simulink model "power_wind_dfig"  (R2016a)
settings: Solver=ode23tb  StartTime=0.0  StopTime=100  FixedStep=1/60  MaxStep=1/60  RelTol=1e-4  AbsTol=1e-3
InitFcn:
  | xInitial = init_power_wind_dfig;
undefined symbols (not defined in the file): b0, D1, D11, Delta, F, find_system, Fnom, gcbh, H, ILd_init, ILq_init, Imax_grid_conv, Init, j, Kd, Ki_dc_reg, Ki_grid_side_cur_reg, Ki_power_reg, Ki_Q, Ki_rotor_side_cur_reg, Ki_volt_reg, Kp, Kp_dc_reg, Kp_grid_side_cur_reg, Kp_power_reg, Kp_Q, Kp_rotor_side_cur_reg, Kp_volt_reg, L_RL, Llr, Lls, p, Pnom, power_A, power_B, power_D, R_RL, Rr, Rs, speed_A, speed_B, speed_C, speed_D, sps_rtmsupport, Vcontrol, Vnom, Wind_On, wo
libraries: powerlib_meascontrol x29, powerlib x27, simulink_extras x5, re_lib x2
(part 1 of 5)
Description:
  | Copyright 2008-2016 The MathWorks, Inc.
settings Model: ExtModeAutoUpdateStatusClock=off  Creator=MathWorks  LastModifiedBy=farhan an
settings DataIOCC: LimitDataPoints=on  LoadInitialState=on  SaveFormat=StructureWithTime  SignalLoggingSaveFormat=ModelDataLogs  SaveOutput=off  InspectSignalLogs=on  SaveTime=off  SignalLoggingName=sigsOut
settings OptimizationCC: ExpressionDepthLimit=2147483647  InitFltsAndDblsToZero=on  EfficientMapNaN2IntZero=off
settings DebuggingCC: UnderspecifiedInitializationDetection=Classic  MergeDetectMultiDrivingBlocksExec=none  CheckExecutionContextPreStartOutputMsg=on  CheckExecutionContextRuntimeOutputMsg=on  SignalResolutionControl=TryResolveAllWithWarning  MultiTaskDSMMsg=warning  MultiTaskCondExecSysMsg=none  FcnCallInpInsideContextMsg=UseLocalSettings  UnconnectedLineMsg=none  StateNameClashWarn=warning  InitInArrayFormatMsg=none
settings HardwareCC: ProdBitPerPointer=32  ProdLargestAtomicFloat=None  ProdIntDivRoundTo=Undefined  ProdEndianess=Unspecified  ProdWordSize=32  ProdHWDeviceType=32-bit Generic  TargetUnknown=on
settings ModelReferenceCC: PropagateSignalLabelsOutOfModel=off
settings GRTTargetCC: CombineOutputUpdateFcns=off  GRTInterface=on
settings ConfigComp: CovModelRefEnable=Off  CovSFcnEnable=off

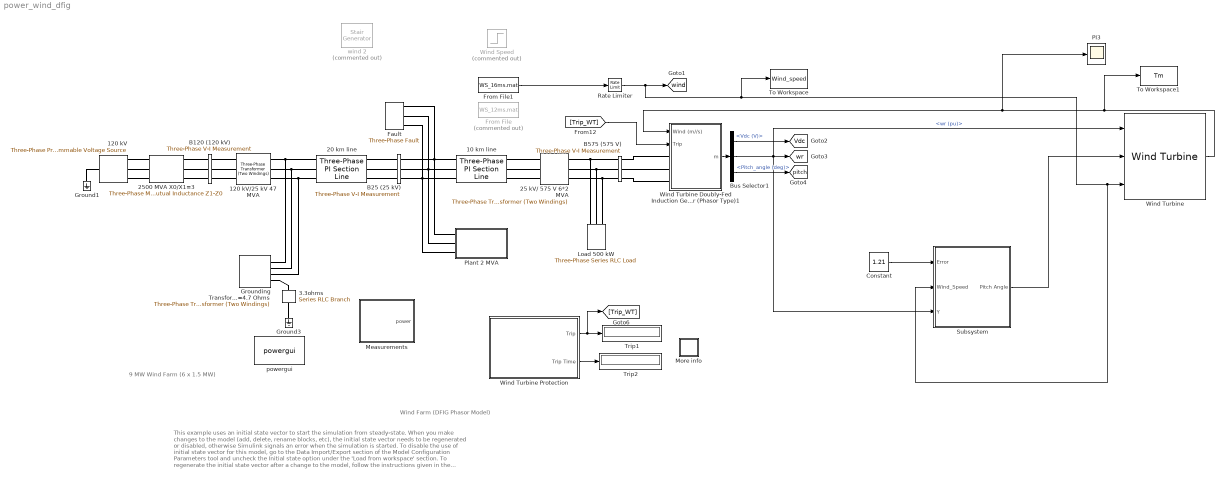
== system power_wind_dfig ==
  note: 9 MW Wind Farm
      | (6 x 1.5 MW)
  note: Wind Farm (DFIG Phasor Model)
  note: This example uses an initial state vector to start the simulation from steady-state. When you make changes to the model (add, delete, rename blocks, etc),
      | the initial state vector needs to be regenerated or disabled, otherwise Simulink signals an error when the simulation is started.
      | To disable the use of initial state vector for this model, go to the Data Import/Export section of the Model Configuration Parameters tool and uncheck the
      | Initial state option under the 'Load from workspace' section.
      | To regenerate the initial state vector after a change to the model, follow the instructions given in the initialization file for this model.
      | Type open('init_power_wind_dfig') at the matlab prompt to view this file.
  10 km line : powerlib/Elements/Three-Phase PI Section Line  LConnTagsString=a|b|c  RConnTagsString=A|B|C  Frequency=60  Resistances=[0.1153 0.413]  Inductances=[1.05e-3 3.32e-3]  Capacitances=[11.33e-009 5.01e-009]  Length=10
  120 kV : powerlib/Electrical Sources/Three-Phase Programmable Voltage Source  PositiveSequence=[120e3 0 60]  VariationEntity=None  VariationType=Step  VariationTypeAlt=Step  VariationStep=-0.15  VariationRate=10  VariationMagnitude=0.3  VariationFrequency=2  VariationTiming=[5 5.5]  VariationPhaseA=off  Amplitudes=[1 0.8 1.2 1.0]  TimeValues=[0 0.1 0.15 0.2]  HarmonicGeneration=off  HarmonicA=[1 -0.1 0 1]  HarmonicB=[2 0.15 35 2]  Timing="[5  5.5]"  BusType=swing  Pref=1e3  Qref=0  Qmin=-inf  Qmax=inf
  120 kV/25 kV 47 MVA : powerlib/Elements/Three-Phase Transformer (Two Windings)  Winding1Connection=Yg  Winding2Connection=Delta (D1)  CoreType=Three single-phase transformers  SetSaturation=off  Hysteresis=off  DataFile='basic_model'  SetInitialFlux=off  Measurements=None  UNITS=pu  NominalPower=[47e6 60 ]  Winding1="[ 120e3  0.08/30   0.08 ]"  Winding2="[ 25e3  0.08/30  0.08]"  Rm=500  Lm=500  L0=0.5  Saturation="[ 0,0  ;  0.005,1.2  ;  1.0,1.4 ]"  InitialFluxes=[ 0.8 , -0.8 , 0.7 ]  MoreParameters=off  BreakLoop=off  DataType=off  TransfoNumber=0
  20 km line : powerlib/Elements/Three-Phase PI Section Line  LConnTagsString=a|b|c  RConnTagsString=A|B|C  Frequency=60  Resistances=[0.1153 0.413]  Inductances=[1.05e-3 3.32e-3]  Capacitances=[11.33e-009 5.01e-009]  Length=20
  25 kV/ 575 V 6*2 MVA : powerlib/Elements/Three-Phase Transformer (Two Windings)  Winding1Connection=Yg  Winding2Connection=Delta (D1)  CoreType=Three single-phase transformers  SetSaturation=off  Hysteresis=off  DataFile='hysteresis'  SetInitialFlux=off  Measurements=None  UNITS=pu  NominalPower="[2e6*6  60]"  Winding1=[25e3 , 0.025/30 , 0.025]  Winding2=[ 575, 0.025/30 , 0.025]  Rm=500  Lm=inf  L0=0.5  Saturation=[ 0,0 ; 0.0024,1.2 ; 1.0,1.52 ]  InitialFluxes=[ 0.8 , -0.8 , 0.7 ]  MoreParameters=off  BreakLoop=off  DataType=off  TransfoNumber=0
  2500 MVA X0/X1=3 : powerlib/Elements/Three-Phase Mutual Inductance Z1-Z0  LConnTagsString=a|b|c  RConnTagsString=A|B|C  PositiveSequence="[0.1  1.0/(2*pi*60)] *120e3^2/2500e6"  ZeroSequence="[0.3  3.0/(2*pi*60)] *120e3^2/2500e6"
  "3.3ohms " : powerlib/Elements/Series RLC Branch  LConnTagsString=__new0  RConnTagsString=__new0  BranchType=R  Resistance=3.3  Inductance=1.0  SetiL0=off  InitialCurrent=0  Capacitance=1.0  Setx0=off  InitialVoltage=0  Measurements=None
  B120 (120 kV) : powerlib/Measurements/Three-Phase V-I Measurement  VoltageMeasurement=phase-to-ground  SetLabelV=on  LabelV=Vabc_B120  Vpu=on  VpuLL=off  CurrentMeasurement=no  SetLabelI=on  LabelI=Iabc_B120  Ipu=off  Pbase=100e6  Vbase=120e3  OutputType=Complex  PhasorSimulation=on  PSBequivalent=0
  B25 (25 kV) : powerlib/Measurements/Three-Phase V-I Measurement  VoltageMeasurement=phase-to-ground  SetLabelV=on  LabelV=Vabc_B25  Vpu=on  VpuLL=off  CurrentMeasurement=yes  SetLabelI=on  LabelI=Iabc_B25  Ipu=on  Pbase=10e6  Vbase=25e3  OutputType=Complex  PhasorSimulation=on  PSBequivalent=0
  B575 (575 V) : powerlib/Measurements/Three-Phase V-I Measurement  VoltageMeasurement=phase-to-ground  SetLabelV=on  LabelV=Vabc_B575  Vpu=on  VpuLL=off  CurrentMeasurement=yes  SetLabelI=on  LabelI=Iabc_B575  Ipu=on  Pbase=6*1.5e6/0.9  Vbase=575  OutputType=Complex  PhasorSimulation=on  PSBequivalent=0
  Bus Selector1 : BusSelector  OutputSignals=Vdc (V),wr (pu),Pitch_angle (deg)
  Constant : Constant  Value=1.21
  Fault : powerlib/Elements/Three-Phase Fault  InitialStates=0  FaultA=off  FaultB=off  FaultC=off  GroundFault=on  SwitchTimes=[ 5 5+9/60]  External=off  SwitchStatus=NaN  FaultResistance=1e-3  GroundResistance=1e-3  SnubberResistance=1e4  SnubberCapacitance=inf  Measurements=None
  From File : FromFile  Commented=on  FileName=WS_12ms.mat  SampleTime=0
  From File1 : FromFile  FileName=WS_16ms.mat  SampleTime=0
  Ground1 : powerlib/Elements/Ground  LConnTagsString=a
  Ground3 : powerlib/Elements/Ground  LConnTagsString=a
  Grounding Transformer X0=4.7 Ohms : powerlib/Elements/Three-Phase Transformer (Two Windings)  Winding1Connection=Yn  Winding2Connection=Delta (D11)  CoreType=Three single-phase transformers  SetSaturation=off  Hysteresis=off  DataFile='basic_model'  SetInitialFlux=off  Measurements=None  UNITS=pu  NominalPower=[100e6 60]  Winding1="[ 25e3  4.7/(25e3^2/100e6)/30    4.7/(25e3^2/100e6)]"  Winding2="[ 25e3  1e-6  0]"  Rm=500  Lm=500  L0=0.5  Saturation="[ 0,0  ;  0.005,1.2  ;  1.0,1.4 ]"  InitialFluxes=[ 0.8 , -0.8 , 0.7 ]  MoreParameters=off  BreakLoop=off  DataType=off  TransfoNumber=0
  Load 500 kW : powerlib/Elements/Three-Phase Series RLC Load  LConnTagsString=A|B|C  Configuration=Y (grounded)  NominalVoltage=575  Vabc=[1e3 1e3 1e3]  Vabcp=[1e3 1e3 1e3]  NominalFrequency=60  UnbalancedPower=off  ActivePower=500e3  InductivePower=0  CapacitivePower=0  Pabc=[10e3 9e3 11e3]  QLabc=[100 90 110]  QCabc=[100 90 110]  Pabcp=[10e3 9e3 11e3]  QLabcp=[100 90 110]  QCabcp=[100 90 110]  Measurements=None  LoadType=constant Z
  Measurements : Subsystem
  More info : Subsystem
      settings: OpenFcn=showdemo(bdroot(gcb))
      mask Display: disp('?')
  PI3 : Scope
  Plant 2 MVA : Subsystem
  Rate Limiter : RateLimiter
  Subsystem : Subsystem
  To Workspace : ToWorkspace  VariableName=Wind_speed  SaveFormat=Timeseries  SampleTime=-1
  To Workspace1 : ToWorkspace  VariableName=Tm  SaveFormat=Timeseries  SampleTime=-1
  Trip1 : Display
  Trip2 : Display
  Wind Speed : Step  Commented=on  Time=5  Before=8  After=14  SampleTime=0
  Wind Turbine : re_lib/Wind Generation/Wind Turbine  Pnom=5e6  Pelec_base=(5e6)/0.9  wind_base=16  P_wind_base=0.9  speed_nom=1.2  pitch_angle=0  c1_c6="[0.51763          116          0.4            5           21     0.006795]"  cp_nom=0.48  lambda_nom=8.1
  Wind Turbine Doubly-Fed Induction Generator (Phasor Type)1 : Subsystem  AncestorBlock=|  DialogController=POWERSYS.PowerSysDialog  LoadFcn=sps_rtmsupport('LoadFcn',gcbh); %find_system(gcs,'FollowLinks', 'on', 'LookUnderMasks', 'all');  StartFcn=sps_rtmsupport('StartFcn',gcbh);  StopFcn=sps_rtmsupport('StopFcn',gcbh);  mask(Wind Turbine Doubly-Fed Induction Generator (Phasor Type)){ExternalTm=on, nom=[5e6/0.9 575 60], sta=[ 0.00706 0.171], rot=[ 0.005 0.156], Lm=2.9, mec=[5.04 0.01 3], init=[0.2 0 0 0 0 0], speed_power=[0 0; 0.24 0.007; 0.36 0.024; 0.6 0.112; 0.96 0.46; 1.2 0.898; 1.5 0.898], Pmec=6*1.5e6, speed_ABCD=[0.7 0.71 1.2 1.21], power_C=0.73, wind_point_C=12, pitch_gain=500, pitch_max=45, pitch_rate=2, Pmax=0.5, Lchoke=[0.15 0.15/100], init_inductor=[0 90], Vdc_nom=1200, capacitor=6*10000e-6, ControlVQ=Voltage regulation, Vref=1.0, ExternalVref=off, Qref=0, ExternalQref=off, Iq_ref=0, ExternalIqref=off, Kpi_volt_reg=[1.25 300], Xs=0.02, Kpi_Q=[0.05 5], Kpi_power_reg=[1 100], Kpi_dc_reg=[0.002 0.05], Kpi_grid_side_cur_reg=[1 100], Kpi_rotor_side_cur_reg=[0.3 8], V_slew_rate=100, Q_slew_rate=100, power_slew_rate=1, current_slew_rate=200}
      | re_lib/Wind Generation/Wind Turbine
      | Doubly-Fed Induction Generator
      | (Phasor Type)
      mask prompts: ExternalTm "External turbine (Tm mechanical torque input)"; nom "Nominal power, line-to-line voltage, frequency [Pn(VA), Vn(Vrms), fn(Hz)]:"; sta "Stator [Rs, Lls] (pu):"; rot "Rotor [Rr', Llr' ] (pu):"; Lm "Magnetizing inductance Lm (pu):"; mec "Inertia constant, friction factor, and pairs of poles [H(s), F(pu),  p ]:"; init "Initial conditions [s,  th(deg),  Is(pu), ph_Is(deg),  Ir(pu),  ph_Ir(deg)]:"; speed_power "Electric power-speed characteristic: [wr1(pu) p1(pu); wr2(pu) p2(pu); ... ]"; Pmec "Nominal wind turbine mechanical output power (W):"; speed_ABCD "Tracking characteristic speeds: [speed_A(pu) ... speed_D(pu)]"; power_C "Power at point C (pu/mechanical power):"; wind_point_C "Wind speed at point C (m/s):"; pitch_gain "Pitch angle controller gain [Kp]:"; pitch_max "Maximum pitch angle (deg):"; pitch_rate "Maximum rate of change of pitch angle (deg/s):"; Pmax "Converter maximum power (pu):"; Lchoke "Grid-side coupling inductor [L (pu) R (pu)]:"; init_inductor "Coupling inductor initial current: [ IL(pu) ph_IL(deg)]"; Vdc_nom "Nominal DC bus voltage (V):"; capacitor "DC bus capacitor (F):"; ControlVQ "Mode:"; Vref "Reference grid voltage Vref (pu):"; ExternalVref "External"; Qref "Generated reactive power Qref (pu):"; ExternalQref "External"; Iq_ref "Grid-side converter generated reactive current reference (Iq_ref) (pu):"; ExternalIqref "External"; Kpi_volt_reg "Grid voltage regulator gains: [Kp Ki]"; Xs "Droop Xs (pu):"; Kpi_Q "Reactive power regulator gains: [Kp Ki]"; Kpi_power_reg "Power regulator gains: [Kp Ki]"; Kpi_dc_reg "DC bus voltage regulator gains: [Kp Ki]"; Kpi_grid_side_cur_reg "Grid-side converter current regulator gains: [Kp Ki]"; Kpi_rotor_side_cur_reg "Rotor-side converter current regulator gains: [Kp Ki]"; V_slew_rate "Maximum rate of change of reference grid voltage (pu/s):"; Q_slew_rate "Maximum rate of change of reference reactive power (pu/s):"; power_slew_rate "Maximum rate of change of reference power (pu/s):"; current_slew_rate "Maximum rate of change of converter  reference currents (pu/s):"
      mask help: Implements a phasor model of a doubly-fed induction generator driven by a wind turbine.
      mask init:
      | [ Pnom, Vnom,Fnom,Rs,Lls,Rr,Llr,H,F,p,mag_IL_init,ph_IL_init,ILd_init,ILq_init,Imax_grid_conv,speed_A,speed_B,speed_C, speed_D,power_A,power_B,power_D,L_RL,R_RL,Kp_volt_reg,Ki_volt_reg,Kp_Q,Ki_Q,Kp_power_reg,Ki_power_reg,Kp_dc_reg,Ki_dc_reg,Kp_grid_side_cur_reg,Ki_grid_side_cur_reg,Kp_rotor_side_cur_reg,Ki_rotor_side_cur_reg,Wind_On,Vcontrol, FACTSroot] = WindTurbineInit( nom,sta,rot,mec,Pmax,Lchoke,init_inductor,ExternalTm,speed_ABCD,power_C,Kpi_volt_reg,Kpi_Q,Kpi_power_reg,Kpi_dc_reg,Kpi_grid_side_cur_reg,Kpi_rotor_side_cur_reg,gcbh,ControlVQ);
      settings: CopyFcn=sps_rtmsupport('CopyFcn',gcbh);  DeleteFcn=sps_rtmsupport('DeleteFcn',gcbh);  UndoDeleteFcn=sps_rtmsupport('UndoDeleteFcn',gcbh);  ModelCloseFcn=sps_rtmsupport('ModelCloseFcn',gcbh);  PreSaveFcn=sps_rtmsupport('PreSaveFcn',gcbh);  PostSaveFcn=sps_rtmsupport('PostSaveFcn',gcbh);  NameChangeFcn=sps_rtmsupport('NameChangeFcn',gcbh);  PreCopyFcn=sps_rtmsupport('PreCopyFcn',gcbh);  OpenFcn=sps_rtmsupport('OpenFcn',gcbh, [1 21,23,25,27]);  CloseFcn=sps_rtmsupport('CloseFcn',gcbh);  PreDeleteFcn=sps_rtmsupport('PreDeleteFcn',gcbh);
      mask Help: helpview(psbhelp)
      mask Callback ExternalTm: WindTurbineCback(gcbh,1);
      mask TypeOptions ControlVQ: Voltage regulation | Var regulation
      mask Callback ControlVQ: WindTurbineCback(gcbh,1);
      mask Callback ExternalVref: WindTurbineCback(gcbh,1);
      mask Callback ExternalQref: WindTurbineCback(gcbh,1);
      mask Callback ExternalIqref: WindTurbineCback(gcbh,1);
      mask DialogControl Display Prompt: Display wind turbine power characteristics
      mask DialogControl Display Callback: WindTurbineDisplay(gcbh);
      mask Display:
      | disp('');
      | image(imread(fullfile(FACTSroot,'eolienne.bmp'),'bmp'))
      | color('white')
      | port_label('LConn',1,'A')
      | port_label('LConn',2,'B')
      | port_label('LConn',3,'C')
      | color('blue')
      | port_label('output',1,'m')
      | port_label('input',1,'Tm')
      | port_label('input',1,'Tm')
      | port_label('input',2,'trip')
  Wind Turbine Protection : Subsystem
      mask Display: disp('Wind\nTurbine\nProtection')
  powergui : powerlib/powergui  Priority=2  SimulationMode=Phasor  SolverType=Tustin  SampleTime=0  frequency=60  SPID=off  DisableSnubberDevices=off  DisableRonSwitches=off  DisableVfSwitches=off  SwTol=0  DisplayEquations=off  Interpol=off  ExternalGateDelay=off  methode=off  Ts=0  FunctionMessages=off  echomessages=off  HookPort=off  EnableUseOfTLC=off  x0status=blocks  frequencyindice=60  Pbase=100e6  ErrMax=1e-4  Iterations=50  UnitsV=kV  UnitsW=MW  buscounter=0  RestoreLinks=warning  ResistiveCurrentMeasurement=off  Frange=[0:2:500]  Ylog=off  Xlog=off  ShowGrid=off  save=off  variable=ZData  structure=0  ZoomFFT=on  StartTime=0.0  cycles=1  DisplayStyle=1  fundamental=60  FreqAxis=off  MaxFrequency=1000  frequencyindicesteady=1  RmsSteady=1  display=off
  wind 2 : powerlib_meascontrol/Pulse & Signal Generators/Stair Generator  Commented=on  t=[0 5 10 15 20 25 30 35 40 45 50 60 70 80 90 100]  e=[8 8 13 13 14 14 12 12 12 13 13 13 12 12 12 12]  Ts=0
  tag scope: Vdc=global, pitch=global, wind=global, wr=global
  wires:
  Bus Selector1/1 -> [Vdc]  "<Vdc (V)>"
  Bus Selector1/2 -> Subsystem/3(Y), [wr], Wind Turbine/1  "<wr (pu)>"
  Wind Turbine Doubly-Fed Induction Generator (Phasor Type)1/1(m) -> Bus Selector1/1
  Wind Turbine Protection/1(Trip) -> [Trip_WT], Trip1/1
  Wind Turbine Protection/2(Trip Time) -> Trip2/1
  Rate Limiter/1 -> To Workspace/1, Subsystem/2(Wind_Speed), Wind Turbine/3, [wind]
  Bus Selector1/3 -> [pitch]  "<Pitch_angle (deg)>"
  [Trip_WT] -> Wind Turbine Doubly-Fed Induction Generator (Phasor Type)1/2(Trip)
  Wind Turbine/1 -> To Workspace1/1, PI3/1, Wind Turbine Doubly-Fed Induction Generator (Phasor Type)1/1("Wind (m//s) ")
  Constant/1 -> Subsystem/1(Error)
  Subsystem/1(Pitch Angle) -> Wind Turbine/2
  From File1/1 -> Rate Limiter/1
  connections:
  Ground1/LConn1 -- 120 kV/LConn1
  120 kV/RConn1 -- 2500 MVA X0/X1=3/LConn1
  120 kV/RConn2 -- 2500 MVA X0/X1=3/LConn2
  120 kV/RConn3 -- 2500 MVA X0/X1=3/LConn3
  "3.3ohms "/RConn1 -- Ground3/LConn1
  Grounding Transformer X0=4.7 Ohms/LConn4 -- "3.3ohms "/LConn1
  B120 (120 kV)/LConn1 -- 2500 MVA X0/X1=3/RConn1
  B120 (120 kV)/LConn2 -- 2500 MVA X0/X1=3/RConn2
  B120 (120 kV)/LConn3 -- 2500 MVA X0/X1=3/RConn3
  120 kV/25 kV 47 MVA/RConn2 -- 20 km line/LConn2 -- Grounding Transformer X0=4.7 Ohms/LConn2
  120 kV/25 kV 47 MVA/RConn3 -- 20 km line/LConn3 -- Grounding Transformer X0=4.7 Ohms/LConn3
  120 kV/25 kV 47 MVA/RConn1 -- 20 km line/LConn1 -- Grounding Transformer X0=4.7 Ohms/LConn1
  20 km line/RConn2 -- B25 (25 kV)/LConn2
  20 km line/RConn3 -- B25 (25 kV)/LConn3
  Fault/LConn1 -- B25 (25 kV)/RConn1 -- Plant 2 MVA/LConn1 -- 10 km line/LConn1
  Fault/LConn2 -- B25 (25 kV)/RConn2 -- Plant 2 MVA/LConn2 -- 10 km line/LConn2
  Fault/LConn3 -- B25 (25 kV)/RConn3 -- Plant 2 MVA/LConn3 -- 10 km line/LConn3
  Load 500 kW/LConn2 -- 25 kV/ 575 V 6*2 MVA/RConn2 -- B575 (575 V)/LConn2
  Load 500 kW/LConn1 -- 25 kV/ 575 V 6*2 MVA/RConn1 -- B575 (575 V)/LConn1
  Load 500 kW/LConn3 -- 25 kV/ 575 V 6*2 MVA/RConn3 -- B575 (575 V)/LConn3
  10 km line/RConn1 -- 25 kV/ 575 V 6*2 MVA/LConn1
  10 km line/RConn2 -- 25 kV/ 575 V 6*2 MVA/LConn2
  10 km line/RConn3 -- 25 kV/ 575 V 6*2 MVA/LConn3
  B120 (120 kV)/RConn1 -- 120 kV/25 kV 47 MVA/LConn1
  B120 (120 kV)/RConn2 -- 120 kV/25 kV 47 MVA/LConn2
  B120 (120 kV)/RConn3 -- 120 kV/25 kV 47 MVA/LConn3
  B25 (25 kV)/LConn1 -- 20 km line/RConn1
  B575 (575 V)/RConn1 -- Wind Turbine Doubly-Fed Induction Generator (Phasor Type)1/LConn1
  B575 (575 V)/RConn2 -- Wind Turbine Doubly-Fed Induction Generator (Phasor Type)1/LConn2
  B575 (575 V)/RConn3 -- Wind Turbine Doubly-Fed Induction Generator (Phasor Type)1/LConn3

== system power_wind_dfig/Measurements ==
  Grid : Scope  NumInputPorts=8
  Grid Data acquisition : Subsystem
  Scope1 : Scope
  To File : ToFile  Filename=pw.mat  SaveFormat=Timeseries
  To Workspace : ToWorkspace  VariableName=Power_pu  SaveFormat=Timeseries  SampleTime=-1
  Wind Turbine : Scope  NumInputPorts=8
  Wind turbine Data acquisition : Subsystem
  power : Outport
  wires:
  Wind turbine Data acquisition/3(P_mean) -> power/1, To Workspace/1, To File/1, Scope1/1, Wind Turbine/3  "Generated P(MW)"
  Grid Data acquisition/1("Vabc_B120 ") -> Grid/1  "Vabc_B120 (pu)"
  Grid Data acquisition/2("Vabc_B25 ") -> Grid/2  "Vabc_B25 (pu)"
  Grid Data acquisition/3("Vabc_B575 ") -> Grid/3  "Vabc_B575 (pu)"
  Grid Data acquisition/4(P_B25) -> Grid/4  "P_B25 (MW)"
  Grid Data acquisition/5(Q_B25) -> Grid/5  "Q_B25 (Mvar)"
  [Vdc] -> Wind Turbine/5  "Vdc (V)"
  [wr] -> Wind Turbine/6  "Speed (pu)"
  Wind turbine Data acquisition/1(V1_B575) -> Wind Turbine/1  "Pos. seq. V1_B575 (pu)"
  Wind turbine Data acquisition/2(I1_B575) -> Wind Turbine/2  "Pos. seq. I1_B575 (pu)"
  Wind turbine Data acquisition/4(Q_mean) -> Wind Turbine/4  "Generated Q(Mvar)"
  Grid Data acquisition/8(Motor_Speed) -> Grid/8  "Motor Speed (pu)"
  Grid Data acquisition/7(I1_Plant) -> Grid/7  "I Plant pos. seq. (pu/2 MVA)"
  Grid Data acquisition/6(V1_Plant) -> Grid/6  "V_Plant 2.3kV pos. seq. (pu)"
  [wind] -> Wind Turbine/7  "Wind speed (m/s)"
  [pitch] -> Wind Turbine/8  "pitch angle (deg)"

== system power_wind_dfig/More info ==

== system power_wind_dfig/Plant 2 MVA ==
  note: Instantaneous AC Overcurrent
  note: AC Overcurrent (positive-sequence)
  note: AC Current Unbalance
  note: AC Undervoltage (positive-sequence)
  note: AC Overvoltage (positive-sequence)
  note: AC Voltage Unbalance (Negative-sequence)
  note: AC Voltage Unbalance (Zero-sequence)
  note: DC Overvoltage
  note: Under Speed
  note: Over Speed
  1.68 MW 0.93 PF 2300 V : powerlib/Machines/Asynchronous Machine pu Units  RotorType=Squirrel-cage  PresetModel=No  MechanicalLoad=Torque Tm  ShowDetailedParameters=on  ReferenceFrame=Rotor  Units=pu  MeasurementBus=off  NominalParameters=[1.68e6/0.93 2300 60]  Stator=[0.0092 0.0717]  Rotor=[0.007 0.0717]  Cage1=[0.01909 0.0397]  Cage2=[0.01909 0.0397]  Lm=4.14  Mechanical=[0.5 0 2]  PolePairs=2  InitialConditions="[ 1e-3,0   0,0,0   0,0,0 ]"  SimulateSaturation=off  Saturation=[ 0 0 ; 0 0 ]  LoadFlowParameters=0  TsPowergui=0  TsBlock=-1  IterativeModel=Forward Euler  IterativeDiscreteModel=Trapezoidal non iterative  Pmec=3e3
  200 kW : powerlib/Elements/Three-Phase Series RLC Load  LConnTagsString=A|B|C  Configuration=Y (grounded)  NominalVoltage=2300  Vabc=[1e3 1e3 1e3]  Vabcp=[1e3 1e3 1e3]  NominalFrequency=60  UnbalancedPower=off  ActivePower=200e3  InductivePower=0  CapacitivePower=0  Pabc=[10e3 9e3 11e3]  QLabc=[100 90 110]  QCabc=[100 90 110]  Pabcp=[10e3 9e3 11e3]  QLabcp=[100 90 110]  QCabcp=[100 90 110]  Measurements=None  LoadType=constant Z
  25/2.3 kV 2.5 MVA : powerlib/Elements/Three-Phase Transformer (Two Windings)  Winding1Connection=Delta (D11)  Winding2Connection=Yn  CoreType=Three single-phase transformers  SetSaturation=off  Hysteresis=off  DataFile='basic_model'  SetInitialFlux=off  Measurements=None  UNITS=pu  NominalPower=[2.5e6 60 ]  Winding1="[ 25e3  0.04/30   0.04 ]"  Winding2="[ 2.3e3  0.04/30  0.04]"  Rm=500  Lm=500  L0=0.5  Saturation="[ 0,0  ;  0.005,1.2  ;  1.0,1.4 ]"  InitialFluxes=[ 0.8 , -0.8 , 0.7 ]  MoreParameters=off  BreakLoop=off  DataType=off  TransfoNumber=0
  265 ohms : powerlib/Elements/Series RLC Branch  LConnTagsString=__new0  RConnTagsString=__new0  BranchType=R  Resistance=265  Inductance=1.0  SetiL0=off  InitialCurrent=0  Capacitance=1.0  Setx0=off  InitialVoltage=0  Measurements=None
  B2300 : powerlib/Measurements/Three-Phase V-I Measurement  VoltageMeasurement=phase-to-ground  SetLabelV=on  LabelV=Vabc_B2300  Vpu=on  VpuLL=off  CurrentMeasurement=yes  SetLabelI=on  LabelI=Iabc_B2300  Ipu=on  Pbase=2.0e6  Vbase=2300  OutputType=Complex  PhasorSimulation=on  PSBequivalent=0
  Bus Selector : BusSelector  OutputSignals=Mechanical.Rotor speed (wm)
  Data Type Conversion : DataTypeConversion  OutDataTypeStr=double  SampleTime=0  SaturateOnIntegerOverflow=on  RndMeth=Zero
  Gain : Gain  Gain=0.9  SaturateOnIntegerOverflow=on  OutDataTypeStr=Inherit: Same as input  ParamDataTypeStr=Inherit: Same as input
  Ground : powerlib/Elements/Ground  LConnTagsString=a
  Ground1 : Ground
  Ground2 : Ground
  Logical Operator : Logic  Operator=NOT  AllPortsSameDT=off
  PF Correction Capacitor 800 kvar : powerlib/Elements/Three-Phase Series RLC Load  LConnTagsString=A|B|C  Configuration=Y (grounded)  NominalVoltage=2300  Vabc=[1e3 1e3 1e3]  Vabcp=[1e3 1e3 1e3]  NominalFrequency=60  UnbalancedPower=off  ActivePower=0  InductivePower=0  CapacitivePower=800e3  Pabc=[10e3 9e3 11e3]  QLabc=[100 90 110]  QCabc=[100 90 110]  Pabcp=[10e3 9e3 11e3]  QLabcp=[100 90 110]  QCabcp=[100 90 110]  Measurements=None  LoadType=constant Z
  Plant & Motor Protection : Subsystem  mask(Protection System){Freq=60, Max_Iinst=10, MaxI1=[ 1.1, 5 ], MaxI2I1=[ 0.4, 0.2], MinMaxV1=[ 0.9, 1.1, 0.2 ], MaxV2V1=[ 0.1, 0.1, 0.3 ], MaxVdc=[ inf, 0 ], MaxSpeed=[ 0.9, 1.1, 1 ], Delay_Protection=1}
      mask prompts: Freq "Fundamental frequency f1 (Hz):"; Max_Iinst "Instantaneous AC Overcurrent (pu):"; MaxI1 "Maximum AC Current [ I1max(pu), Delay(s) ]:"; MaxI2I1 "Maximum AC Current Unbalance [ I2/I1max(pu), Delay(s) ]"; MinMaxV1 "AC Under/Over Voltage [ V1min(pu), V1max(pu), Delay(s) ]:"; MaxV2V1 "Maximum Voltage Unbalance [ V2/V1max(pu), V0/V1max(pu), Delay(s)]:"; MaxVdc "Maximum DC Voltage  [ Vmax(V), Delay(s) ]:"; MaxSpeed "Under/Over Speed [ Speedmin (pu), Speedmax (pu), Delay(s)]:"; Delay_Protection "Start time for protection system (s):"
      mask help:
      | Protection type:
      | 1.    Instantaneous AC Overcurrent
      | 2.    AC Overcurrent (positive-sequence)
      | 3.    AC Current Unbalance
      | 4.    AC Undervoltage (positive-sequence)
      | 5.    AC Overvoltage (positive-sequence)
      | 6.    AC Voltage Unbalance (Negative-sequence)
      | 7.    AC Voltage Unbalance (Zero-sequence)
      | 8.    DC Overvoltage
      | 9.    Under Speed
      | 10.  Over Speed
      mask init:
      | a=exp(2*pi*j/3);
      | a2=a^2;
      | Max_I1=MaxI1(1);
      | Delay_I1=MaxI1(2);
      | Max_I2_I1=MaxI2I1(1);
      | Delay_I2_I1=MaxI2I1(2);
      | Min_V1=MinMaxV1(1);
      | Max_V1=MinMaxV1(2);
      | Delay_V1=MinMaxV1(3);
      | Max_V2_V1=MaxV2V1(1);
      | Max_V0_V1=MaxV2V1(2);
      | Delay_V2_V1=MaxV2V1(3);
      | Max_Vdc=MaxVdc(1);
      | Delay_Vdc=MaxVdc(2);
      | Min_Speed=MaxSpeed(1);
      | Max_Speed=MaxSpeed(2);
      | Delay_Speed=MaxSpeed(3);
  Three-Phase Breaker : powerlib/Elements/Three-Phase Breaker  InitialState=closed  SwitchA=on  SwitchB=on  SwitchC=on  SwitchTimes="[4/60  10/60]"  External=on  BreakerResistance=0.001  SnubberResistance=inf  SnubberCapacitance=inf  Measurements=None
  Trip1 : Display
  TripData : Display
  wm^2 : Fcn  Expr=u(1)^2
  A : PMIOPort  Port=1  Side=Left
  B : PMIOPort  Port=2  Side=Left
  C : PMIOPort  Port=3  Side=Left
  tag scope: MotorSpeed=global
  wires:
  1.68 MW 0.93 PF 2300 V/1 -> Bus Selector/1
  Bus Selector/1 -> wm^2/1, [MotorSpeed]  "<Rotor speed (wm)>"
  wm^2/1 -> Gain/1
  [Vabc_B2300] -> Plant & Motor Protection/1(Vabc (pu))
  [Iabc_B2300] -> Plant & Motor Protection/2(Iabc (pu))
  Ground1/1 -> Plant & Motor Protection/3(Vdc (V))
  Ground2/1 -> Plant & Motor Protection/4(Reset)
  [MotorSpeed] -> Plant & Motor Protection/5(Speed (pu))
  Plant & Motor Protection/1(Trip) -> Logical Operator/1
  [Trip_Plant] -> Three-Phase Breaker/1
  Plant & Motor Protection/2(TripTime) -> Trip1/1
  Plant & Motor Protection/3(TripStatus) -> TripData/1
  Data Type Conversion/1 -> [Trip_Plant]
  Logical Operator/1 -> Data Type Conversion/1
  Gain/1 -> 1.68 MW 0.93 PF 2300 V/1
  connections:
  265 ohms/LConn1 -- 25/2.3 kV 2.5 MVA/RConn4
  Ground/LConn1 -- 265 ohms/RConn1
  A/RConn1 -- 25/2.3 kV 2.5 MVA/LConn1
  B/RConn1 -- 25/2.3 kV 2.5 MVA/LConn2
  C/RConn1 -- 25/2.3 kV 2.5 MVA/LConn3
  25/2.3 kV 2.5 MVA/RConn1 -- B2300/LConn1 -- PF Correction Capacitor 800 kvar/LConn1
  25/2.3 kV 2.5 MVA/RConn2 -- B2300/LConn2 -- PF Correction Capacitor 800 kvar/LConn2
  B2300/LConn3 -- 25/2.3 kV 2.5 MVA/RConn3 -- PF Correction Capacitor 800 kvar/LConn3
  B2300/RConn1 -- Three-Phase Breaker/LConn1
  B2300/RConn2 -- Three-Phase Breaker/LConn2
  B2300/RConn3 -- Three-Phase Breaker/LConn3
  Three-Phase Breaker/RConn1 -- 1.68 MW 0.93 PF 2300 V/LConn1 -- 200 kW/LConn1
  Three-Phase Breaker/RConn2 -- 1.68 MW 0.93 PF 2300 V/LConn2 -- 200 kW/LConn2
  Three-Phase Breaker/RConn3 -- 1.68 MW 0.93 PF 2300 V/LConn3 -- 200 kW/LConn3

== system power_wind_dfig/Subsystem ==
  Error : Inport
  Wind_Speed : Inport  Port=2
  Y : Inport  Port=3
  0-pitch_max : Saturate  UpperLimit=45  LowerLimit=0
  Demux : Demux  Outputs=3
  Gain1 : Gain  Gain=Kp
  Gain2 : Gain  Gain=10
  Gain3 : Gain  Gain=1/b0
  Gain4 : Gain  Gain=1000
  Gain5 : Gain  Gain=Kd
  Gain6 : Gain  Gain=1010
  "LESO " : StateSpace  A=[-3*wo 1 0;-3*wo^2 0 1; -wo^3 0 0]  B=[0 3*wo ;b0 3*wo^2 ; 0 wo^3 ]  C=eye(3)  D=[0,0;0,0;0,0]  X0=0
  Mux : Mux  Inputs=2
  Scope : Scope  NumInputPorts=2
  Scope{1..4} (4 alike) : Scope
  Sum : Sum  Inputs=|-+
  Sum2 : Sum  Inputs=|+-
  Sum3 : Sum  Inputs=|+--
  To Workspace : ToWorkspace  VariableName=Pitch  SaveFormat=Timeseries  SampleTime=-1
  To Workspace1 : ToWorkspace  VariableName=wr  SaveFormat=Timeseries  SampleTime=-1
  Transfer Fcn : TransferFcn  Denominator=[0.5 1]
  Pitch Angle : Outport
  wires:
  0-pitch_max/1 -> Gain6/1, Gain4/1, Pitch Angle/1
  Sum2/1 -> Transfer Fcn/1
  Transfer Fcn/1 -> 0-pitch_max/1, Sum2/2
  "LESO "/1 -> Demux/1
  Sum/1 -> Gain1/1
  Gain1/1 -> Sum3/1
  Demux/2 -> Scope3/1, Gain5/1
  Error/1 -> Sum/1
  Sum3/1 -> Gain3/1
  Mux/1 -> "LESO "/1
  Y/1 -> Mux/2
  Gain4/1 -> Gain2/1, Scope/1
  Gain3/1 -> Mux/1, Sum2/1
  Demux/3 -> Scope4/1, Sum3/3
  Gain5/1 -> Sum3/2
  Wind_Speed/1 -> Scope/2
  Gain2/1 -> Scope2/1
  Demux/1 -> Sum/2, To Workspace1/1, Scope1/1
  Gain6/1 -> To Workspace/1

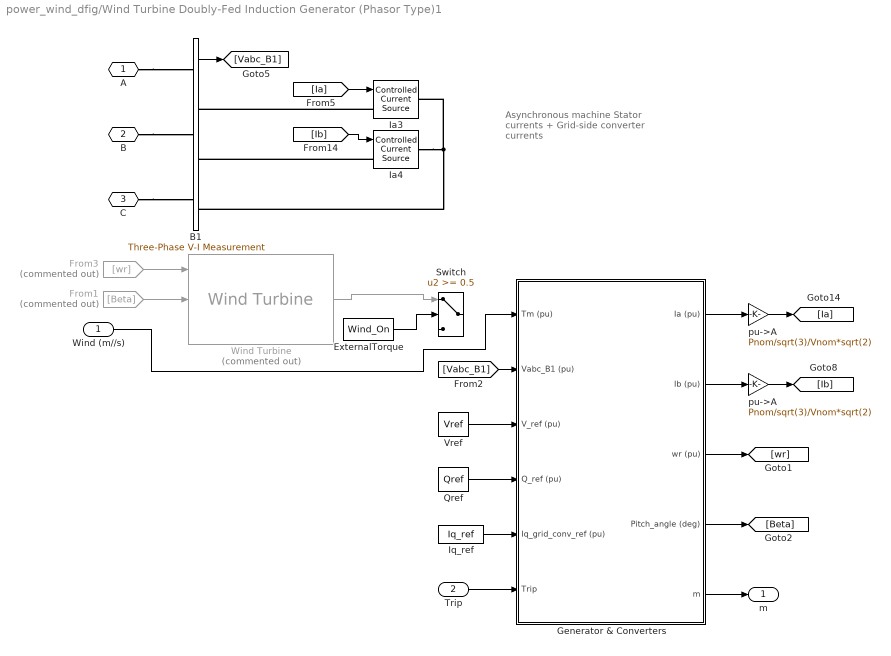
== system power_wind_dfig/Wind Turbine Doubly-Fed Induction Generator (Phasor Type)1 ==
  note: Asynchronous machine
      | Stator currents
      | +
      | Grid-side converter
      | currents
  "Wind (m//s) " : Inport
  Trip : Inport  Port=2
  B1 : powerlib/Measurements/Three-Phase V-I Measurement  VoltageMeasurement=phase-to-ground  SetLabelV=off  LabelV=Vabc_B1  Vpu=on  VpuLL=off  CurrentMeasurement=no  SetLabelI=off  LabelI=Iabc_Beol  Ipu=off  Pbase=Pnom  Vbase=Vnom  OutputType=Complex  PhasorSimulation=on  PSBequivalent=0
  ExternalTorque : Constant  Value=Wind_On
  From1 : From  Commented=on  GotoTag=Beta
      settings: CloseFcn=tagdialog Close
  From3 : From  Commented=on  GotoTag=wr
      settings: CloseFcn=tagdialog Close
  Generator & Converters : Subsystem
  Ia3 : powerlib/Electrical Sources/Controlled Current Source  Description=source block  Initialize=off  Source_Type=AC  Amplitude=0  Phase=0  Frequency=0  Measurements=None
  Ia4 : powerlib/Electrical Sources/Controlled Current Source  Description=source block  Initialize=off  Source_Type=AC  Amplitude=0  Phase=0  Frequency=0  Measurements=None
  "Iq_ref " : Constant  Value=Iq_ref
  "Qref " : Constant  Value=Qref
  Switch : Switch  Threshold=0.5  SaturateOnIntegerOverflow=on
  "Vref " : Constant  Value=Vref
  Wind Turbine : re_lib/Wind Generation/Wind Turbine  Commented=on  Pnom=Pmec  Pelec_base=Pnom  wind_base=wind_point_C  P_wind_base=power_C  speed_nom=speed_C  pitch_angle=0  c1_c6="[0.51763          116          0.4            5           21     0.006795]"  cp_nom=0.48  lambda_nom=8.1
  "pu->A " : Gain  Gain=Pnom/sqrt(3)/Vnom*sqrt(2)  SaturateOnIntegerOverflow=on  OutDataTypeStr=Inherit: Same as input  ParamDataTypeStr=Inherit: Same as input
  "pu->A  " : Gain  Gain=Pnom/sqrt(3)/Vnom*sqrt(2)  SaturateOnIntegerOverflow=on  OutDataTypeStr=Inherit: Same as input  ParamDataTypeStr=Inherit: Same as input
  A : PMIOPort  Port=1  Side=Left
  B : PMIOPort  Port=2  Side=Left
  C : PMIOPort  Port=3  Side=Left
  m : Outport
  wires:
  Generator & Converters/4(Pitch_angle (deg)) -> [Beta]
  From1/1 -> Wind Turbine/2
  Trip/1 -> Generator & Converters/6(Trip)
  [Ib] -> Ia4/1
  [Ia] -> Ia3/1
  "Vref "/1 -> Generator & Converters/3(V_ref (pu))
  "Iq_ref "/1 -> Generator & Converters/5(Iq_grid_conv_ref (pu))
  "Qref "/1 -> Generator & Converters/4(Q_ref (pu))
  Generator & Converters/5(m) -> m/1
  Wind Turbine/1 -> Switch/1
  From3/1 -> Wind Turbine/1
  Generator & Converters/2(Ib (pu)) -> "pu->A  "/1
  ExternalTorque/1 -> Switch/2
  Generator & Converters/3(wr (pu)) -> [wr]
  B1/1 -> [Vabc_B1]
  "pu->A "/1 -> [Ia]
  "pu->A  "/1 -> [Ib]
  Generator & Converters/1(Ia (pu)) -> "pu->A "/1
  [Vabc_B1] -> Generator & Converters/2(Vabc_B1 (pu))
  "Wind (m//s) "/1 -> Generator & Converters/1(Tm (pu))
  connections:
  Ia3/LConn1 -- B1/RConn1
  A/RConn1 -- B1/LConn1
  Ia4/LConn1 -- B1/RConn2
  Ia4/RConn1 -- Ia3/RConn1 -- B1/RConn3
  C/RConn1 -- B1/LConn3
  B/RConn1 -- B1/LConn2

== system power_wind_dfig/Wind Turbine Protection ==
  note: Instantaneous AC Overcurrent
  note: AC Overcurrent (positive-sequence)
  note: AC Current Unbalance
  note: AC Undervoltage (positive-sequence)
  note: AC Overvoltage (positive-sequence)
  note: AC Voltage Unbalance (Negative-sequence)
  note: AC Voltage Unbalance (Zero-sequence)
  note: DC Overvoltage
  note: Under Speed
  note: Over Speed
  Ground2 : Ground
  Protection System : Subsystem  mask(Protection System){Freq=60, Max_Iinst=10, MaxI1=[ 1.1, 5 ], MaxI2I1=[ 0.4, 0.2], MinMaxV1=[ 0.75, 1.1, 0.1 ], MaxV2V1=[ 0.05, 0.05, 0.2 ], MaxVdc=[ 1900, 0.001 ], MaxSpeed=[ 0.3, 1.5, 5 ], Delay_Protection=5}
      mask prompts: Freq "Fundamental frequency f1 (Hz):"; Max_Iinst "Instantaneous AC Overcurrent (pu):"; MaxI1 "Maximum AC Current [ I1max(pu), Delay(s) ]:"; MaxI2I1 "Maximum AC Current Unbalance [ I2/I1max(pu), Delay(s) ]"; MinMaxV1 "AC Under/Over Voltage [ V1min(pu), V1max(pu), Delay(s) ]:"; MaxV2V1 "Maximum Voltage Unbalance [ V2/V1max(pu), V0/V1max(pu), Delay(s)]:"; MaxVdc "Maximum DC Voltage  [ Vmax(V), Delay(s) ]:"; MaxSpeed "Under/Over Speed [ Speedmin (pu), Speedmax (pu), Delay(s)]:"; Delay_Protection "Start time for protection system (s):"
      mask help:
      | Protection type:
      | 1.    Instantaneous AC Overcurrent
      | 2.    AC Overcurrent (positive-sequence)
      | 3.    AC Current Unbalance
      | 4.    AC Undervoltage (positive-sequence)
      | 5.    AC Overvoltage (positive-sequence)
      | 6.    AC Voltage Unbalance (Negative-sequence)
      | 7.    AC Voltage Unbalance (Zero-sequence)
      | 8.    DC Overvoltage
      | 9.    Under Speed
      | 10.  Over Speed
      mask init: same as power_wind_dfig/Plant 2 MVA/Plant & Motor Protection
  TripData : Display
  Trip : Outport
  Trip Time : Outport  Port=2
  wires:
  Ground2/1 -> Protection System/4(Reset)
  Protection System/3(TripStatus) -> TripData/1
  [Vabc_B575] -> Protection System/1(Vabc (pu))
  [Vdc] -> Protection System/3(Vdc (V))
  [wr] -> Protection System/5(Speed (pu))
  [Iabc_B575] -> Protection System/2(Iabc (pu))
  Protection System/1(Trip) -> Trip/1
  Protection System/2(TripTime) -> Trip Time/1

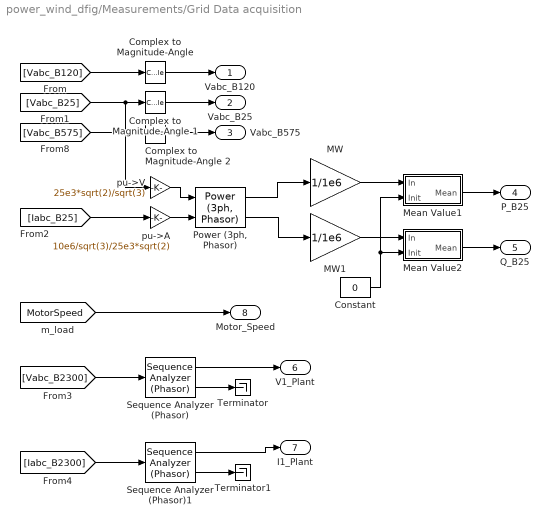
== system power_wind_dfig/Measurements/Grid Data acquisition ==
  "Complex to Magnitude-Angle " : ComplexToMagnitudeAngle  Output=Magnitude
  Complex to Magnitude-Angle 1 : ComplexToMagnitudeAngle  Output=Magnitude
  Complex to Magnitude-Angle 2 : ComplexToMagnitudeAngle  Output=Magnitude
  Constant : Constant  Value=0
  MW : Gain  Gain=1/1e6  SaturateOnIntegerOverflow=on  OutDataTypeStr=Inherit: Same as input  ParamDataTypeStr=Inherit: Same as input
  MW1 : Gain  Gain=1/1e6  SaturateOnIntegerOverflow=on  OutDataTypeStr=Inherit: Same as input  ParamDataTypeStr=Inherit: Same as input
  Mean Value1 : Subsystem  mask(Mean value){Period=1/60}
      mask prompts: Period "Averaging period (s):"
      mask help: This block uses the running window averaging technique to compute the mean value of the input signal over the specified period.
  Mean Value2 : Subsystem  mask(Mean value){Period=1/60}
      mask prompts: Period "Averaging period (s):"
      mask help: This block uses the running window averaging technique to compute the mean value of the input signal over the specified period.
  "Power (3ph, Phasor)" : powerlib_meascontrol/Measurements/Power (3ph, Phasor)
  Sequence Analyzer (Phasor) : powerlib_meascontrol/Measurements/Sequence Analyzer (Phasor)  seq=Positive
  Sequence Analyzer (Phasor)1 : powerlib_meascontrol/Measurements/Sequence Analyzer (Phasor)  seq=Positive
  Terminator : Terminator
  Terminator1 : Terminator
  pu->A : Gain  Gain=10e6/sqrt(3)/25e3*sqrt(2)  SaturateOnIntegerOverflow=on  OutDataTypeStr=Inherit: Same as input  ParamDataTypeStr=Inherit: Same as input
  pu->V : Gain  Gain=25e3*sqrt(2)/sqrt(3)  SaturateOnIntegerOverflow=on  OutDataTypeStr=Inherit: Same as input  ParamDataTypeStr=Inherit: Same as input
  "Vabc_B120 " : Outport
  "Vabc_B25 " : Outport  Port=2
  "Vabc_B575 " : Outport  Port=3
  P_B25 : Outport  Port=4
  Q_B25 : Outport  Port=5
  V1_Plant : Outport  Port=6
  I1_Plant : Outport  Port=7
  Motor_Speed : Outport  Port=8
  wires:
  pu->A/1 -> "Power (3ph, Phasor)"/2
  pu->V/1 -> "Power (3ph, Phasor)"/1
  "Complex to Magnitude-Angle "/1 -> "Vabc_B120 "/1
  [Vabc_B120] -> "Complex to Magnitude-Angle "/1
  Complex to Magnitude-Angle 1/1 -> "Vabc_B25 "/1
  [Vabc_B25] -> Complex to Magnitude-Angle 1/1, pu->V/1
  Complex to Magnitude-Angle 2/1 -> "Vabc_B575 "/1
  [Vabc_B575] -> Complex to Magnitude-Angle 2/1
  [Iabc_B25] -> pu->A/1
  Constant/1 -> Mean Value1/2(Init), Mean Value2/2(Init)
  Mean Value1/1(Mean) -> P_B25/1
  Mean Value2/1(Mean) -> Q_B25/1
  [MotorSpeed] -> Motor_Speed/1
  [Vabc_B2300] -> Sequence Analyzer (Phasor)/1
  Sequence Analyzer (Phasor)/1 -> V1_Plant/1
  Sequence Analyzer (Phasor)/2 -> Terminator/1
  [Iabc_B2300] -> Sequence Analyzer (Phasor)1/1
  Sequence Analyzer (Phasor)1/1 -> I1_Plant/1
  Sequence Analyzer (Phasor)1/2 -> Terminator1/1
  MW/1 -> Mean Value1/1(In)
  MW1/1 -> Mean Value2/1(In)
  "Power (3ph, Phasor)"/1 -> MW/1
  "Power (3ph, Phasor)"/2 -> MW1/1

== system power_wind_dfig/Measurements/Wind turbine Data acquisition ==
  Constant : Constant  Value=0
  Gain3 : Gain  Gain=1/3  SaturateOnIntegerOverflow=on  OutDataTypeStr=Inherit: Same as input  ParamDataTypeStr=Inherit: Same as input
  Gain4 : Gain  Gain=1/3  SaturateOnIntegerOverflow=on  OutDataTypeStr=Inherit: Same as input  ParamDataTypeStr=Inherit: Same as input
  MW : Gain  Gain=-1/1e6  SaturateOnIntegerOverflow=on  OutDataTypeStr=Inherit: Same as input  ParamDataTypeStr=Inherit: Same as input
  MW1 : Gain  Gain=-1/1e6  SaturateOnIntegerOverflow=on  OutDataTypeStr=Inherit: Same as input  ParamDataTypeStr=Inherit: Same as input
  Mean Value1 : Subsystem  mask(Mean value){Period=1/60}
      mask prompts: Period "Averaging period (s):"
      mask help: This block uses the running window averaging technique to compute the mean value of the input signal over the specified period.
  Mean Value2 : Subsystem  mask(Mean value){Period=1/60}
      mask prompts: Period "Averaging period (s):"
      mask help: This block uses the running window averaging technique to compute the mean value of the input signal over the specified period.
  "Power (3ph, Phasor)" : powerlib_meascontrol/Measurements/Power (3ph, Phasor)
  Sum : Sum  Inputs=1  SaturateOnIntegerOverflow=on  InputSameDT=on  OutDataTypeStr=Inherit: Same as first input
  Sum1 : Sum  Inputs=1  SaturateOnIntegerOverflow=on  InputSameDT=on  OutDataTypeStr=Inherit: Same as first input
  abc_to_pos : Gain  Gain=[1 exp(j*2*pi/3) exp(-j*2*pi/3)]  SaturateOnIntegerOverflow=on  OutDataTypeStr=Inherit: Same as input  ParamDataTypeStr=Inherit: Same as input
  abc_to_pos1 : Gain  Gain=[1 exp(j*2*pi/3) exp(-j*2*pi/3)]  SaturateOnIntegerOverflow=on  OutDataTypeStr=Inherit: Same as input  ParamDataTypeStr=Inherit: Same as input
  "magnitude positive seq. " : Subsystem
  magnitude positivie seq : Subsystem
  pu->A : Gain  Gain=(6*1.5e6/0.9)/sqrt(3)/575*sqrt(2)  SaturateOnIntegerOverflow=on  OutDataTypeStr=Inherit: Same as input  ParamDataTypeStr=Inherit: Same as input
  pu->V : Gain  Gain=575*sqrt(2)/sqrt(3)  SaturateOnIntegerOverflow=on  OutDataTypeStr=Inherit: Same as input  ParamDataTypeStr=Inherit: Same as input
  V1_B575 : Outport
  I1_B575 : Outport  Port=2
  P_mean : Outport  Port=3
  Q_mean : Outport  Port=4
  wires:
  [Iabc_B575] -> pu->A/1, abc_to_pos1/1
  [Vabc_B575] -> pu->V/1, abc_to_pos/1
  pu->A/1 -> "Power (3ph, Phasor)"/2
  pu->V/1 -> "Power (3ph, Phasor)"/1
  MW/1 -> Mean Value1/1(In)
  MW1/1 -> Mean Value2/1(In)
  "magnitude positive seq. "/1(Out1) -> I1_B575/1
  magnitude positivie seq/1(Out1) -> V1_B575/1
  abc_to_pos/1 -> Sum/1
  Sum/1 -> Gain3/1
  Sum1/1 -> Gain4/1
  Gain3/1 -> magnitude positivie seq/1(In1)
  abc_to_pos1/1 -> Sum1/1
  Gain4/1 -> "magnitude positive seq. "/1(In1)
  Mean Value1/1(Mean) -> P_mean/1
  Mean Value2/1(Mean) -> Q_mean/1
  Constant/1 -> Mean Value1/2(Init), Mean Value2/2(Init)
  "Power (3ph, Phasor)"/1 -> MW/1
  "Power (3ph, Phasor)"/2 -> MW1/1

== system power_wind_dfig/Plant 2 MVA/Plant & Motor Protection ==
  Vabc (pu) : Inport  PortDimensions=3
  Iabc (pu) : Inport  Port=2  PortDimensions=3
  Vdc (V) : Inport  Port=3  PortDimensions=1
  Reset : Inport  Port=4  PortDimensions=1
  Speed (pu) : Inport  Port=5  PortDimensions=1
  AC Current Protection : Subsystem
  AC Voltage Protection : Subsystem
  Bistable1 : powerlib_meascontrol/Logic/Bistable  Qpriority=Set  ic=0  Ts=0
  Clock : Clock
  Constant : Constant  Value=Delay_Protection
  DC Voltage Protection : Subsystem
  Decoding : Subsystem
  Encoding : Subsystem
  Logical Operator : Logic  Operator=OR  Inputs=10  AllPortsSameDT=off
  Logical Operator1 : Logic  AllPortsSameDT=off
  Logical Operator2 : Logic  Operator=NOT  AllPortsSameDT=off
  Logical Operator3 : Logic  AllPortsSameDT=off
  Memory : Memory  InheritSampleTime=on
  Memory1 : Memory  InheritSampleTime=on
  Monostable1 : powerlib_meascontrol/Logic/Monostable  EdgeDetect=Rising  PulseDuration=1e-9  ic=0  Ts=0
  Relational Operator10 : RelationalOperator
  Sample & Hold : Subsystem  DialogController=POWERSYS.PowerSysDialog  mask(Sample & Hold){ic=0}
      mask prompts: ic "Initial condition:"
      mask help: The output follows input 1 (In) as long as input 2 (S) is TRUE (1) . The output is held when input 2 becomes FALSE (0). The output initial value is specified by the parameter "Initial condition".
      mask init:
      | power_initmask();
      mask Help: This block is part of a subset of blocks in the Extras library that does not have documentation associated with it, other than the block mask description.
      mask Display: disp('S/H')
  Sample & Hold1 : Subsystem  DialogController=POWERSYS.PowerSysDialog  mask(Sample & Hold){ic=0}
      mask prompts: ic "Initial condition:"
      mask help: The output follows input 1 (In) as long as input 2 (S) is TRUE (1) . The output is held when input 2 becomes FALSE (0). The output initial value is specified by the parameter "Initial condition".
      mask init:
      | power_initmask();
      mask Help: This block is part of a subset of blocks in the Extras library that does not have documentation associated with it, other than the block mask description.
      mask Display: disp('S/H')
  Terminator : Terminator
  Under/Over Speed Protection : Subsystem
  Trip : Outport
  TripTime : Outport  Port=2
  TripStatus : Outport  Port=3
  wires:
  Memory1/1 -> Trip/1
  Vdc (V)/1 -> DC Voltage Protection/1(Vdc)
  DC Voltage Protection/1(MaxVdc) -> Logical Operator/8, Encoding/8(In8)
  Logical Operator2/1 -> Logical Operator3/1
  Reset/1 -> Logical Operator3/2
  Logical Operator3/1 -> Bistable1/2
  Logical Operator1/1 -> Bistable1/1, Logical Operator2/1
  Encoding/1(Code) -> Sample & Hold/1(In)
  Bistable1/1 -> Memory/1
  Memory/1 -> Monostable1/1, Memory1/1
  Bistable1/2 -> Terminator/1
  Sample & Hold/1("   ") -> Decoding/1(Code)
  Decoding/1(Out) -> TripStatus/1
  Iabc (pu)/1 -> AC Current Protection/1(abc)
  Vabc (pu)/1 -> AC Voltage Protection/1(abc)
  AC Current Protection/1(MaxIinst) -> Logical Operator/1, Encoding/1(In1)
  AC Current Protection/2(MaxI1) -> Logical Operator/2, Encoding/2(In2)
  AC Current Protection/3(MaxI2I1) -> Logical Operator/3, Encoding/3(In3)
  AC Voltage Protection/1(MinV1) -> Logical Operator/4, Encoding/4(In4)
  AC Voltage Protection/2(MaxV1) -> Logical Operator/5, Encoding/5(In5)
  AC Voltage Protection/3(MaxV2V1) -> Logical Operator/6, Encoding/6(In6)
  AC Voltage Protection/4(MaxV0V1) -> Logical Operator/7, Encoding/7(In7)
  Sample & Hold1/1("   ") -> TripTime/1
  Monostable1/1 -> Sample & Hold/2(S), Sample & Hold1/2(S)
  Constant/1 -> Relational Operator10/2
  Clock/1 -> Relational Operator10/1, Sample & Hold1/1(In)
  Logical Operator/1 -> Logical Operator1/1
  Relational Operator10/1 -> Logical Operator1/2
  Under/Over Speed Protection/1(MinSpeed) -> Logical Operator/9, Encoding/9(In9)
  Under/Over Speed Protection/2(MaxSpeed) -> Logical Operator/10, Encoding/10(In10)
  Speed (pu)/1 -> Under/Over Speed Protection/1(Speed)
